simulink library "lcm_lib"  (Simulink 8.2)
settings: Solver=ode45  StartTime=0.0  StopTime=10.0  RelTol=1e-3
PostLoadFcn:
  | , if any(exist('dsrtsu_mdlpostloadfcn', 'file') == [2, 3, 6]), try dsrtsu_mdlpostloadfcn('Execute', bdroot); catch fprintf('Error in PostLoadFcn (dsrtsu_mdlpostloadfcn) for model "%s":\n %s\n', bdroot, lasterr); end, end,
undefined symbols (not defined in the file or in its folder): splitTargetAddress
libraries: simulink x3, dspnetwork x2, rtiethernetlib x2
settings Model: DSRTSU_INTERNAL_RTI_VER=440  DSRTSU_INTERNAL_RTI_TYPE=rti1007  DSRTSU_INTERNAL_RTIFLEXRAYCONFIG=70  DSRTSU_INTERNAL_RTIFPGA=30  Creator=dschoordsch  LastModifiedBy=pkarlss6

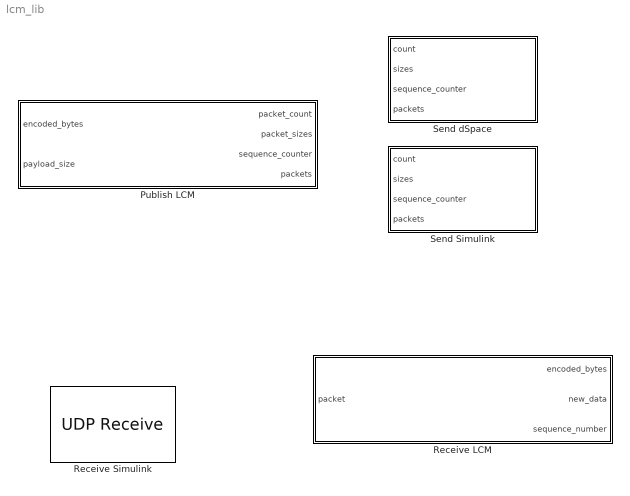
== system lcm_lib ==
  Publish LCM : Subsystem  mask(Publish){channelNameIn='FsmObjectSensorData', maxPayloadSize=5600, maxUdpPacketSize=1400}
      mask prompts: channelNameIn "Channel Name"; maxPayloadSize "Maximal Payload Size"; maxUdpPacketSize "Maximal UDP Packet Size"
      mask help:
      | This will publish the supplied encoded byte array according to the LCM multicast protocol. The publisher and subscriber must use the same port and channel name. It is adviced to use the generated TYPE_encode functions to generate the input byte array.
      |
      | If the maximum payload size wrapped in LCM is smaller than the maximum packet size, the maximum packet size is reduced.
      mask init:
      | if ~ischar(channelNameIn)
      |     error('Channel name must be a string');
      | end
      | channelName = cast(channelNameIn, 'uint8');
      | 
      | %maxUdpPacketSize = 65507;
      | fragmentedHeaderSize = 20;
      | smallHeaderSize = 8;
      | channelNameSize = string_encodedSize_nohash(channelName);
      | 
      | smallMessageSize = maxPayloadSize+smallHeaderSize+channelNameSize;
      | 
      | if smallMessageSize <= maxUdpPacketSize
      |     maxPacketCount = 1;
      |     maxPacketSize = smallMessageSize;
      | else
      |     maxPacketCount = ceil((maxPayloadSize+channelNameSize) / (maxUdpPacketSize-fragmentedHeaderSize));
      |     maxPacketSize = maxUdpPacketSize;
      | end
      mask Help:
      | Channel Name:
      | Identifier of the message stated within quotations marks, used by the receiver to filter out the message from other messages. Example: 'Channel 1'
      | 
      | Maximal packet size:
      | The total payload size of one message, excluding LCM overhead. Used to set the buffer sizes. Example: 5600.
      | 
      | Maximal packet size:
      | This size determines if and how to split one message into smaller fragments. Example: 1400.
      mask Display:
      | fprintf('Publish to\n%s\nPayload/packet size: %i/%i\nMax message count: %i', channelNameIn, maxPayloadSize, maxPacketSize, maxPacketCount);
      | 
      | port_label('output', 4, 'packets');
      | port_label('output', 3, 'seq counter');
      | port_label('output', 2, 'sizes');
      | port_label('output', 1, 'count');
      | port_label('input', 1, 'payload');
      | port_label('input', 2, 'size');
  Receive LCM : Subsystem  mask{channelNameIn='EgoVehicleData', maxPayloadSize=5600, maxUdpPacketSize=65507}
      mask prompts: channelNameIn "Channel Name"; maxPayloadSize "Maximal Payload Size"; maxUdpPacketSize "Maximal Udp Packet Size (leave at 1400 for ethernet)"
      mask init:
      | if ~ischar(channelNameIn)
      |     error('Channel name must be a string');
      | end
      | channelName = cast(channelNameIn, 'uint8');
      | 
      | %maxUdpPacketSize = 65507;
      | fragmentedHeaderSize = 20;
      | smallHeaderSize = 8;
      | channelNameSize = string_encodedSize_nohash(channelName);
      | 
      | smallMessageSize = maxPayloadSize+smallHeaderSize+channelNameSize;
      | 
      | if smallMessageSize <= maxUdpPacketSize
      |     maxPacketCount = 1;
      |     maxPacketSize = maxUdpPacketSize;%smallMessageSize;
      | else
      |     maxPacketCount = ceil((maxPayloadSize+channelNameSize) / (maxUdpPacketSize-fragmentedHeaderSize));
      |     maxPacketSize = maxUdpPacketSize;
      | end
      mask Display:
      | fprintf('Recieve from\n%s\nPayload/packet size: %i/%i\nMax message count: %i', channelNameIn, maxPayloadSize, maxUdpPacketSize, maxPacketCount);
      | 
      | port_label('output', 3, 'sequence number');
      | port_label('output', 2, 'new data');
      | port_label('output', 1, 'encoded bytes');
      | port_label('input', 1, 'packet');
  Receive Simulink : dspnetwork/UDP Receive  localURL='0.0.0.0'  localPort=7667  remoteURL='0.0.0.0'  remotePort=-1  recvBufferSize=74200  dims=1400  signalDatatype=uint8  isVarSize=on  showBlockingTime=off  blockingTime=0  sampletime=0.001
  Send Simulink : Subsystem  TreatAsAtomicUnit=on  SystemSampleTime=.005  mask{targetAddress='127.0.0.1', targetPort=7667}
      mask prompts: targetAddress "Target address"; targetPort "Target port"
      mask Display: fprintf('IP: %s\nPort: %d', targetAddress, targetPort)
  Send dSpace : Subsystem  TreatAsAtomicUnit=on  SystemSampleTime=0.005  mask{targetAddress='169.254.145.241', targetPort=7667}
      mask prompts: targetAddress "Target address"; targetPort "Target port"
      mask Display: fprintf('IP: %s\nPort: %d', targetAddress, targetPort)

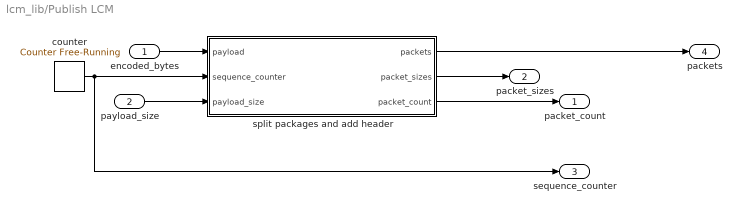
== system lcm_lib/Publish LCM ==
  encoded_bytes : Inport  OutDataTypeStr=uint8
  payload_size : Inport  Port=2
  counter : simulink/Sources/Counter Free-Running  NumBits=32  tsamp=-1
  split packages and add header : MATLAB Function  TreatAsAtomicUnit=on
  packet_count : Outport
  packet_sizes : Outport  Port=2
  sequence_counter : Outport  Port=3
  packets : Outport  Port=4
  wires:
  counter/1 -> split packages and add header/2(sequence_counter), sequence_counter/1
  encoded_bytes/1 -> split packages and add header/1(payload)
  split packages and add header/2(packet_sizes) -> packet_sizes/1
  split packages and add header/3(packet_count) -> packet_count/1
  split packages and add header/1(packets) -> packets/1
  payload_size/1 -> split packages and add header/3(payload_size)

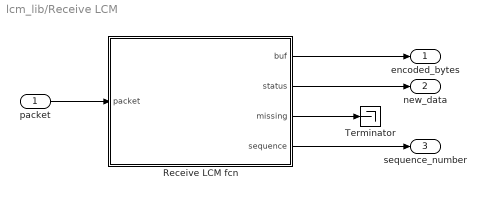
== system lcm_lib/Receive LCM ==
  packet : Inport
  Receive LCM fcn : MATLAB Function  TreatAsAtomicUnit=on
  Terminator : Terminator
  encoded_bytes : Outport
  new_data : Outport  Port=2
  sequence_number : Outport  Port=3
  wires:
  Receive LCM fcn/3(missing) -> Terminator/1
  Receive LCM fcn/2(status) -> new_data/1
  Receive LCM fcn/4(sequence) -> sequence_number/1
  Receive LCM fcn/1(buf) -> encoded_bytes/1
  packet/1 -> Receive LCM fcn/1(packet)

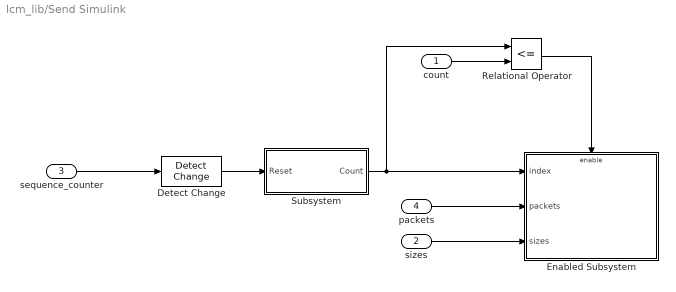
== system lcm_lib/Send Simulink ==
  count : Inport  OutDataTypeStr=uint16  PortDimensions=1
  sizes : Inport  Port=2
  sequence_counter : Inport  Port=3
  packets : Inport  Port=4
  Detect Change : simulink/Logic and Bit Operations/Detect Change  vinit=0  InputProcessing=Inherited  OutDataTypeStr=uint8
  Enabled Subsystem : Subsystem  TreatAsAtomicUnit=on
  Relational Operator : RelationalOperator  Operator=<=  OutDataTypeStr=boolean
  Subsystem : Subsystem
  wires:
  count/1 -> Relational Operator/2
  Relational Operator/1 -> Enabled Subsystem/Enable
  Subsystem/1(Count) -> Relational Operator/1, Enabled Subsystem/1(index)
  Detect Change/1 -> Subsystem/1(Reset)
  sequence_counter/1 -> Detect Change/1
  sizes/1 -> Enabled Subsystem/3(sizes)
  packets/1 -> Enabled Subsystem/2(packets)

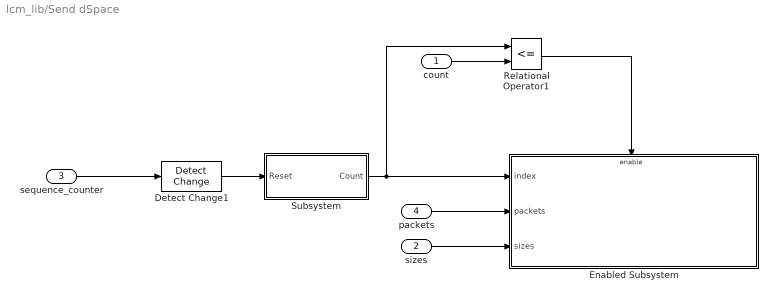
== system lcm_lib/Send dSpace ==
  count : Inport  OutDataTypeStr=uint16  PortDimensions=1
  sizes : Inport  Port=2
  sequence_counter : Inport  Port=3
  packets : Inport  Port=4
  Detect Change1 : simulink/Logic and Bit Operations/Detect Change  vinit=0  InputProcessing=Inherited  OutDataTypeStr=uint8
  Enabled Subsystem : Subsystem
  Relational Operator1 : RelationalOperator  Operator=<=  OutDataTypeStr=boolean
  Subsystem : Subsystem
  wires:
  sequence_counter/1 -> Detect Change1/1
  Detect Change1/1 -> Subsystem/1(Reset)
  Subsystem/1(Count) -> Relational Operator1/1, Enabled Subsystem/1(index)
  Relational Operator1/1 -> Enabled Subsystem/Enable
  count/1 -> Relational Operator1/2
  packets/1 -> Enabled Subsystem/2(packets)
  sizes/1 -> Enabled Subsystem/3(sizes)

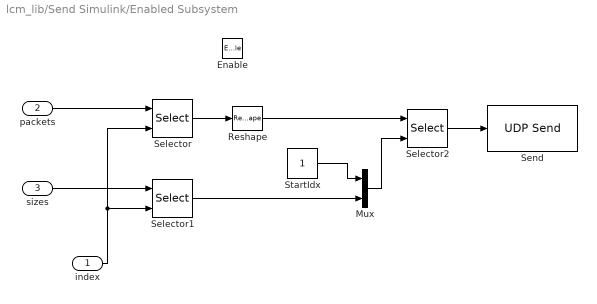
== system lcm_lib/Send Simulink/Enabled Subsystem ==
  index : Inport
  packets : Inport  Port=2
  sizes : Inport  Port=3
  Enable : EnablePort  PropagateVarSize=During execution
  Mux : Mux  Inputs=2
  Reshape : Reshape
  Selector : Selector  NumberOfDimensions=2  InputPortWidth=3  IndexOptions=Select all,Index vector (port)  Indices=[1 3],1  OutputSizes=1,1
  Selector1 : Selector  NumberOfDimensions=2  InputPortWidth=1  IndexOptions=Index vector (dialog),Index vector (port)  Indices=1,1  OutputSizes=1,1
  Selector2 : Selector  IndexOptions=Starting and ending indices (port)  Indices=[1 3]  OutputSizes=1
  Send : dspnetwork/UDP Send  remoteURL=targetAddress  remotePort=targetPort  localURL='127.0.0.1'  localPortSource=Automatically determine  localPort=-1  sampletime=-1  separateLengthPort=0
  StartIdx : Constant  OutDataTypeStr=uint32
  wires:
  index/1 -> Selector1/2, Selector/2
  sizes/1 -> Selector1/1
  packets/1 -> Selector/1
  Selector1/1 -> Mux/2
  Selector/1 -> Reshape/1
  Reshape/1 -> Selector2/1
  Selector2/1 -> Send/1
  Mux/1 -> Selector2/2
  StartIdx/1 -> Mux/1

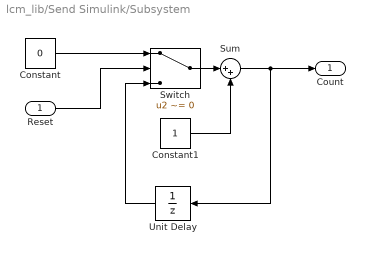
== system lcm_lib/Send Simulink/Subsystem ==
  Reset : Inport
  Constant : Constant  Value=0
  Constant1 : Constant
  Sum : Sum  Inputs=|++
  Switch : Switch  Criteria=u2 ~= 0
  Unit Delay : UnitDelay  SampleTime=-1
  Count : Outport
  wires:
  Sum/1 -> Unit Delay/1, Count/1
  Switch/1 -> Sum/1
  Unit Delay/1 -> Switch/3
  Reset/1 -> Switch/2
  Constant/1 -> Switch/1
  Constant1/1 -> Sum/2

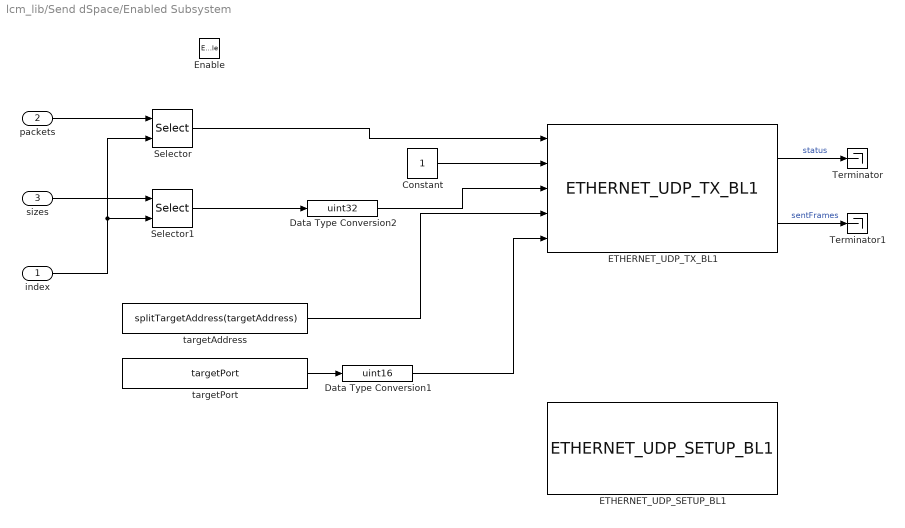
== system lcm_lib/Send dSpace/Enabled Subsystem ==
  index : Inport
  packets : Inport  Port=2
  sizes : Inport  Port=3
  Enable : EnablePort
  Constant : Constant  OutDataTypeStr=boolean
  Data Type Conversion1 : DataTypeConversion  OutDataTypeStr=uint16
  Data Type Conversion2 : DataTypeConversion  OutDataTypeStr=uint32
  ETHERNET_UDP_SETUP_BL1 : rtiethernetlib/ETHERNET_UDP_SETUP_BL1  DSProperties=struct('RTI',struct('Version',uint32(1),'BlockType',struct('isSLSource',uint8(1),'isSLSink',uint8(1),'isHWSource',uint8(0),'isHWSink',uint8(0),'isSetup',uint8(0),'isInline',uint8(1),'isNonInline',uint8(0),'isInterrupt',uint8(0),'isChannelwise',uint8(0)),'IOBoardType','DSETHERNET','UnitType','UDP','Identifier','SETUPUDP','DialogType','ML','BlockSet','RTIETHERNET','SlaveProcessor','NONE'))  RTIBlockInterface=struct('OutputPortsWidth',int32(2),'OutputPortsActive',0,'OutputPortsName',{{['RX Dropped Frames']}},'OutputPortsDataType',{{'SS_DOUBLE'}},'InputPortsWidth',int32([4 1]),'InputPortsActive',int32([0 0]),'InputPortsName',{{['RX Remote IP Filter'],['RX Remote Port Filter']}},'InputPortsDataType',{{'SS_UINT8','SS_UINT16'}},'RWork',{{{'RX_DROPPED_FRAMES',uint32(2)}}},'InitLevel',3,'IconTransparency','on','BlockDisplay',{{['Ethernet UDP/IP\nSetup\n\nSocket ID: 3'],'center'}},'DialogFcn','rtiethernetsetupudpgui','BlockName',struct('Token',{{'ETHERNET_UDP_SETUP_BL1'}}))  RTIBlockParameters=struct('SocketId',{{3,'OFF',[]}},'AcceptAnyRxRemoteIp',{{1,'OFF',[0 1]}},'RxRemoteIpNum1',{{'0','OFF',[0 255]}},'RxRemoteIpNum2',{{'0','OFF',[0 255]}},'RxRemoteIpNum3',{{'0','OFF',[0 255]}},'RxRemoteIpNum4',{{'0','OFF',[0 255]}},'EnableDynamicRxRemoteIpFilter',{{0,'OFF',[0 1]}},'AcceptAnyRxRemotePort',{{1,'OFF',[0 1]}},'RxRemotePort',{{'49002','OFF',[1 65535]}},'EnableDynamicRxRemotePortFilter',{{0,'OFF',[0 1]}},'TxRemoteIpNum1',{{'169','OFF',[0 255]}},'TxRemoteIpNum2',{{'254','OFF',[0 255]}},'TxRemoteIpNum3',{{'245','OFF',[0 255]}},'TxRemoteIpNum4',{{'241','OFF',[0 255]}},'TxRemotePort',{{'7667','OFF',[1 65535]}},'SpecifyLocalPort',{{1,'OFF',[0 1]}},'LocalPort',{{'57667','OFF',[1 65535]}},'InterruptMode',{{0,'OFF',[0 1]}},'RxDroppedFramesOutPortMode',{{0,'OFF',[0 1]}},'RemoteIpNumCheck',{{0,'OFF',[0 1]}},'RemotePortCheck',{{0,'OFF',[0 1]}},'LocalPortCheck',{{1,'OFF',[0 1]}},'DHCPserverModeEnabled',{{0,'OFF',[0 1]}},'TLCFileName',{{'rtiethernetsetupudp','OFF',[]}})  RTISFcnParameters=struct('SocketId','double','AcceptAnyRxRemoteIp','int32','RxRemoteIpNum1','uint8','RxRemoteIpNum2','uint8','RxRemoteIpNum3','uint8','RxRemoteIpNum4','uint8','EnableDynamicRxRemoteIpFilter','int32','AcceptAnyRxRemotePort','int32','RxRemotePort','uint16','EnableDynamicRxRemotePortFilter','int32','TxRemoteIpNum1','uint8','TxRemoteIpNum2','uint8','TxRemoteIpNum3','uint8','TxRemoteIpNum4','uint8','TxRemotePort','uint16','SpecifyLocalPort','int32','LocalPort','uint16','InterruptMode','int32','RxDroppedFramesOutPortMode','int32','DHCPserverModeEnabled','int32','TLCFileName','char')  RTIBlockParaDefault=struct('SocketId',-1,'AcceptAnyRxRemoteIp',1,'RxRemoteIpNum1',0,'RxRemoteIpNum2',0,'RxRemoteIpNum3',0,'RxRemoteIpNum4',0,'EnableDynamicRxRemoteIpFilter',0,'AcceptAnyRxRemotePort',1,'RxRemotePort',49002,'EnableDynamicRxRemotePortFilter',0,'TxRemoteIpNum1',0,'TxRemoteIpNum2',0,'TxRemoteIpNum3',0,'TxRemoteIpNum4',0,'TxRemotePort',49002,'SpecifyLocalPort',0,'LocalPort',49001,'InterruptMode',0,'RxDroppedFramesOutPortMode',0,'RemoteIpNumCheck',0,'RemotePortCheck',0,'LocalPortCheck',0,'DHCPserverModeEnabled',0,'TLCFileName','rtiethernetsetupudp')
  ETHERNET_UDP_TX_BL1 : rtiethernetlib/ETHERNET_UDP_TX_BL1  DSProperties=struct('RTI',struct('Version',uint32(1),'BlockType',struct('isSLSource',uint8(1),'isSLSink',uint8(1),'isHWSource',uint8(0),'isHWSink',uint8(1),'isSetup',uint8(0),'isInline',uint8(1),'isNonInline',uint8(0),'isInterrupt',uint8(0),'isChannelwise',uint8(0)),'IOBoardType','DSETHERNET','UnitType','UDP','Identifier','TXUDP','DialogType','ML','BlockSet','RTIETHERNET','SlaveProcessor','NONE'))  RTIBlockInterface=struct('OutputPortsWidth',int32([1 1]),'OutputPortsActive',[1 1],'OutputPortsName',{{'Status',['Sent Frames']}},'OutputPortsDataType',{{'SS_UINT32','SS_DOUBLE'}},'InputPortsWidth',int32([1400 1 1 4 1]),'InputPortsActive',[1 1 1 1 1],'InputPortsName',{{'Data','Enable',['Bytes to Send'],['Remote IP'],['Remote Port']}},'InputPortsDataType',{{'SS_UINT8','SS_BOOLEAN','SS_UINT32','SS_UINT8','SS_UINT16'}},'RWork',{{{'SENT_FRAMES',uint32(1)}}},'InitLevel',3,'IconTransparency','on','BlockDisplay',{{['Ethernet UDP/IP\nTX\n\nSocket ID: 3'],'center'}},'DialogFcn','rtiethernettxudpgui','BlockName',struct('Token',{{'ETHERNET_UDP_TX_BL1'}}))  RTIBlockParameters=struct('SocketIdIndex',{{5,'OFF',[1 5]}},'SocketId',{{3,'OFF',[-1 inf]}},'RemoteIp',{{['<NOT AVAILABLE>'],'OFF',[]}},'RemotePort',{{['<NOT AVAILABLE>'],'OFF',[]}},'LocalPort',{{['<NOT AVAILABLE>'],'OFF',[]}},'EnableDynamicRemoteIp',{{1,'OFF',[0 1]}},'EnableDynamicRemotePort',{{1,'OFF',[0 1]}},'FrameSize',{{'1400','OFF',[1 65507]}},'EnableVariableFrameSize',{{1,'OFF',[0 1]}},'SentFramesOutPortMode',{{1,'OFF',[0 1]}},'RemoteIpNum',{{[0 0 0 0],'OFF',[0 255]}},'RemotePortNum',{{0,'OFF',[0 65535]}},'TLCFileName',{{'rtiethernettxudp','OFF',[]}})  RTISFcnParameters=struct('SocketIdIndex','int32','SocketId','double','EnableDynamicRemoteIp','int32','EnableDynamicRemotePort','int32','FrameSize','uint16','EnableVariableFrameSize','int32','SentFramesOutPortMode','int32','RemoteIpNum','uint8','RemotePortNum','uint16','TLCFileName','char')  RTIBlockParaDefault=struct('SocketIdIndex',1,'SocketId',-1,'RemoteIp',['<NOT AVAILABLE>'],'RemotePort',['<NOT AVAILABLE>'],'LocalPort',['<NOT AVAILABLE>'],'EnableDynamicRemoteIp',0,'EnableDynamicRemotePort',0,'FrameSize',1024,'EnableVariableFrameSize',0,'SentFramesOutPortMode',1,'RemoteIpNum',[0 0 0 0],'RemotePortNum',0,'TLCFileName','rtiethernettxudp')
  Selector : Selector  NumberOfDimensions=2  InputPortWidth=3  IndexOptions=Select all,Index vector (port)  Indices=[1 3],1  OutputSizes=1,1
  Selector1 : Selector  NumberOfDimensions=2  InputPortWidth=1  IndexOptions=Index vector (dialog),Index vector (port)  Indices=1,1  OutputSizes=1,1
  Terminator : Terminator
  Terminator1 : Terminator
  targetAddress : Constant  Value=splitTargetAddress(targetAddress)
  targetPort : Constant  Value=targetPort
  wires:
  Data Type Conversion1/1 -> ETHERNET_UDP_TX_BL1/5
  targetAddress/1 -> ETHERNET_UDP_TX_BL1/4
  Data Type Conversion2/1 -> ETHERNET_UDP_TX_BL1/3
  targetPort/1 -> Data Type Conversion1/1
  ETHERNET_UDP_TX_BL1/2 -> Terminator1/1  "sentFrames"
  ETHERNET_UDP_TX_BL1/1 -> Terminator/1  "status"
  Constant/1 -> ETHERNET_UDP_TX_BL1/2
  packets/1 -> Selector/1
  sizes/1 -> Selector1/1
  index/1 -> Selector/2, Selector1/2
  Selector/1 -> ETHERNET_UDP_TX_BL1/1
  Selector1/1 -> Data Type Conversion2/1

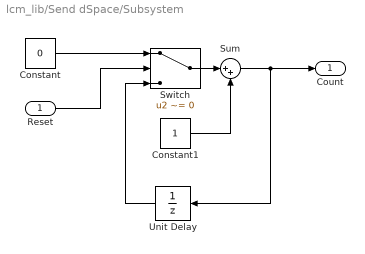
== system lcm_lib/Send dSpace/Subsystem ==
  Reset : Inport
  Constant : Constant  Value=0
  Constant1 : Constant
  Sum : Sum  Inputs=|++
  Switch : Switch  Criteria=u2 ~= 0
  Unit Delay : UnitDelay  SampleTime=-1
  Count : Outport
  wires:
  Sum/1 -> Unit Delay/1, Count/1
  Switch/1 -> Sum/1
  Unit Delay/1 -> Switch/3
  Reset/1 -> Switch/2
  Constant/1 -> Switch/1
  Constant1/1 -> Sum/2

== matlab function Receive LCM/Receive LCM fcn ==
  data: packet input double size=[maxPacketSize, 1]; buf output double size=[maxPacketSize* maxPacketCount, 1]; status output double size=1; missing output double; sequence output double; channelName parameter double; maxPacketSize parameter double size=1; maxPacketCount parameter double size=1
%param status 1 - message received, 0 - only partially received, -1 - error
function [buf, status, missing, sequence] = receive_bundle(packet, channelName, maxPacketSize, maxPacketCount)
%#codegen

[buf, pos, missing, sequence] = receiveMessage(packet, channelName, maxPacketSize, maxPacketCount);
status = 0;
if pos > 0
    status = 1;
end

== matlab function Publish LCM/split packages and add header ==
  data: payload input uint8 size=maxPayloadSize; packets output uint8 size=[maxPacketSize, maxPacketCount]; sequence_counter input uint32 size=1; payload_size input uint32; packet_sizes output uint32 size=[1, maxPacketCount]; maxPacketSize parameter double size=1; maxPacketCount parameter double size=1; channelName parameter double; packet_count output uint16 size=1
function [packets, packet_sizes, packet_count] = header(payload, sequence_counter, payload_size, maxPacketSize, maxPacketCount, channelName)
%#eml
%#codegen
[packets, packet_sizes, packet_count] = prepareMessage(payload, sequence_counter, channelName, payload_size, maxPacketSize, maxPacketCount);
